simulink library "aerosimlib"  (Simulink 5.0)
values from neighbouring files (symbols this model uses):
  stdatm = [0 100 200 300 400 500 600 700 800 900 1000 1100 ... (4305 elements, 861x5)]    [stdatm.mat]
undefined symbols (not defined in the file or in its folder): AlphaBnd, b, BetaBnd, CDda, CDde, CDdf, CDdr, CDM, CDmin, CGempty, CGgross, CL0, CLa, CLalphadot, Clbeta, Clda, CLde, CLdf, Cldr, CLM, CLmind, Clp, CLq, Clr, Cm0, Cma, Cmalphadot, Cmde, Cmdf, CmM, Cmq, Cnbeta, Cnda, Cndr, Cnp, Cnr, CP, CT, CYbeta, CYda, CYdr, CYp, CYr, Displacement, dmy, Engine, EulerIni, FuelFlow, FuelIni, J, Jempty, Jeng, Jgross, Jprop, MAC, MAP, MAPLim, MassIni, MaxPower, mempty ... (+25)
libraries: aerosimlib x350, simulink3 x41
(part 8 of 10)

== system aerosimlib/FlightGear-Compatible/Complete Aircraft/CESSNA-182/Equations of Motion ==
  note: Inputs
  note: Outputs
  Accel : Inport  PortDimensions=[3 1]
  Moment : Inport  Port=2  PortDimensions=[3 1]
  Inertia : Inport  Port=3  PortDimensions=[4 1]
  Rearth : Inport  Port=4  PortDimensions=[2 1]
  Gravity : Inport  Port=5  PortDimensions=1
  AConGnd : Inport  Port=6  PortDimensions=1
  RST : Inport  Port=7  PortDimensions=1
  Angular Rate : aerosimlib/Equations of Motion/Geodetic-Frame EOM/Angular Rate  RatesIni=RatesIni
  Attitude (Quaternions) : aerosimlib/Equations of Motion/Body-Frame EOM/Kinematics (Quaternions)  QuaternionsIni=QuaternionsIni
  Body-Inertial DCM From Quaternions : aerosimlib/Transformations/Body-Inertial DCM From Quaternions
  Demux : Demux  Outputs=2
  Euler Angles From Quaternions : aerosimlib/Transformations/Euler Angles From Quaternions
  Position : aerosimlib/Equations of Motion/Geodetic-Frame EOM/Position  PositionIni=PositionIni
  Product : Product  Multiplication=Matrix(*)  SaturateOnIntegerOverflow=on  InputSameDT=on
  Velocity : aerosimlib/Equations of Motion/Geodetic-Frame EOM/Velocity  VelocitiesIni=VelocitiesIni
  VelB : Outport
  VelNED : Outport  Port=2
  Rates : Outport  Port=3
  Quaternions : Outport  Port=4
  Pos : Outport  Port=5
  DCM : Outport  Port=6
  Euler : Outport  Port=7
  Ang Acc : Outport  Port=8
  wires:
  Attitude (Quaternions)/1 -> Quaternions/1, Euler Angles From Quaternions/1, Body-Inertial DCM From Quaternions/1
  Position/1 -> Velocity/1, Angular Rate/3, Pos/1
  Position/2 -> Velocity/2, Angular Rate/4
  Velocity/1 -> Product/2, Position/1, VelNED/1
  Demux/1 -> Position/2
  Demux/2 -> Position/3
  Rearth/1 -> Demux/1
  Gravity/1 -> Velocity/5
  RST/1 -> Velocity/6, Position/5, Angular Rate/6, Attitude (Quaternions)/2
  Angular Rate/1 -> Rates/1, Attitude (Quaternions)/1
  Moment/1 -> Angular Rate/2
  Inertia/1 -> Angular Rate/1
  Body-Inertial DCM From Quaternions/1 -> Angular Rate/5, Velocity/4, Product/1, DCM/1
  AConGnd/1 -> Position/4
  Accel/1 -> Velocity/3
  Product/1 -> VelB/1
  Angular Rate/2 -> Ang Acc/1
  Euler Angles From Quaternions/1 -> Euler/1

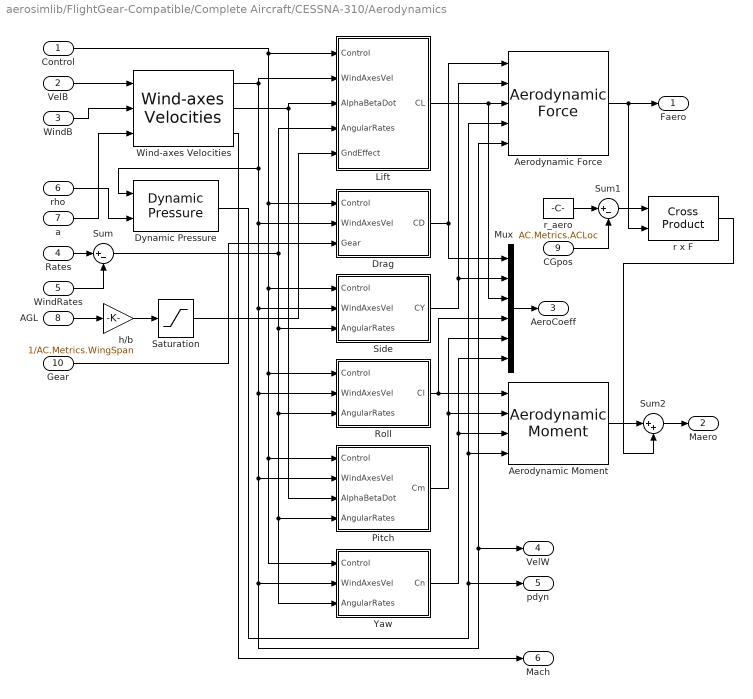
== system aerosimlib/FlightGear-Compatible/Complete Aircraft/CESSNA-310/Aerodynamics ==
  Control : Inport  PortDimensions=[4 1]
  VelB : Inport  Port=2  PortDimensions=[3 1]
  WindB : Inport  Port=3  PortDimensions=[3 1]
  Rates : Inport  Port=4  PortDimensions=[3 1]
  WindRates : Inport  Port=5  PortDimensions=[3 1]
  rho : Inport  Port=6  PortDimensions=1
  a : Inport  Port=7  PortDimensions=1
  AGL : Inport  Port=8  PortDimensions=1
  CGpos : Inport  Port=9  PortDimensions=[3 1]
  Gear : Inport  Port=10  PortDimensions=1
  Aerodynamic Force : aerosimlib/Aerodynamics/Aerodynamic Force  S=AC.Metrics.WingArea
  Aerodynamic Moment : aerosimlib/Aerodynamics/Aerodynamic Moment  c=AC.Metrics.WingChord  b=AC.Metrics.WingSpan  S=AC.Metrics.WingArea
  Drag : Subsystem
  Dynamic Pressure : aerosimlib/Aerodynamics/Dynamic Pressure
  Lift : Subsystem
  Mux : Mux  Inputs=6
  Pitch : Subsystem
  Roll : Subsystem
  Saturation : Saturate  UpperLimit=1  LowerLimit=0
  Side : Subsystem
  Sum : Sum  Inputs=|+-  SaturateOnIntegerOverflow=on  InputSameDT=on
  Sum1 : Sum  Inputs=|+-  SaturateOnIntegerOverflow=on  InputSameDT=on
  Sum2 : Sum  Inputs=|++  SaturateOnIntegerOverflow=on  InputSameDT=on
  Wind-axes Velocities : aerosimlib/Aerodynamics/Wind-axes Velocities  Vabnd=[0 1000]  betabnd=[-1 1]  alphabnd=AC.Aerodynamics.AlphaLim
  Yaw : Subsystem
  h/b : Gain  Gain=1/AC.Metrics.WingSpan  SaturateOnIntegerOverflow=on
  r x F : aerosimlib/Math/Cross Product
  r_aero : Constant  Value=AC.Metrics.ACLoc
  Faero : Outport
  Maero : Outport  Port=2
  AeroCoeff : Outport  Port=3
  VelW : Outport  Port=4
  pdyn : Outport  Port=5
  Mach : Outport  Port=6
  wires:
  Gear/1 -> Drag/3(Gear)
  r x F/1 -> Sum2/2
  Sum2/1 -> Maero/1
  Aerodynamic Moment/1 -> Sum2/1
  Sum1/1 -> r x F/1
  r_aero/1 -> Sum1/1
  CGpos/1 -> Sum1/2
  Rates/1 -> Sum/1
  Sum/1 -> Yaw/3(AngularRates), Pitch/4(AngularRates), Roll/3(AngularRates), Side/3(AngularRates), Lift/4(AngularRates)
  WindRates/1 -> Sum/2
  Saturation/1 -> Lift/5(GndEffect)
  AGL/1 -> h/b/1
  h/b/1 -> Saturation/1
  Wind-axes Velocities/3 -> Mach/1
  Aerodynamic Force/1 -> r x F/2, Faero/1
  Yaw/1(Cn) -> Mux/6, Aerodynamic Moment/3
  Pitch/1(Cm) -> Mux/5, Aerodynamic Moment/2
  Roll/1(Cl) -> Mux/4, Aerodynamic Moment/1
  Dynamic Pressure/1 -> pdyn/1, Aerodynamic Moment/4, Aerodynamic Force/4
  Side/1(CY) -> Mux/2, Aerodynamic Force/2
  Drag/1(CD) -> Mux/1, Aerodynamic Force/1
  Lift/1(CL) -> Mux/3, Aerodynamic Force/3
  Wind-axes Velocities/2 -> Lift/3(AlphaBetaDot), Pitch/3(AlphaBetaDot)
  Control/1 -> Pitch/1(Control), Yaw/1(Control), Roll/1(Control), Side/1(Control), Drag/1(Control), Lift/1(Control)
  Wind-axes Velocities/1 -> Lift/2(WindAxesVel), VelW/1, Aerodynamic Force/5, Yaw/2(WindAxesVel), Pitch/2(WindAxesVel), Roll/2(WindAxesVel), Side/2(WindAxesVel), Drag/2(WindAxesVel), Dynamic Pressure/1
  rho/1 -> Dynamic Pressure/2
  a/1 -> Wind-axes Velocities/3
  WindB/1 -> Wind-axes Velocities/2
  VelB/1 -> Wind-axes Velocities/1
  Mux/1 -> AeroCoeff/1

== system aerosimlib/FlightGear-Compatible/Complete Aircraft/CESSNA-310/Aircraft Inertia ==
  FuelFlow : Inport
  RST : Inport  Port=2
  1/Ntank : Gain  Gain=1/length(AC.Propulsion.Tank)  SaturateOnIntegerOverflow=on
  Empty Aircraft : aerosimlib/FlightGear-Compatible/Inertia/Empty Aircraft  Metrics=AC.Metrics
  Left Inner Tank : aerosimlib/FlightGear-Compatible/Propulsion/Tank/Fuel Tank  MassIni=FuelIni(3)  Tank=AC.Propulsion.Tank{3}
  Left Outer Tank : aerosimlib/FlightGear-Compatible/Propulsion/Tank/Fuel Tank  MassIni=FuelIni(1)  Tank=AC.Propulsion.Tank{1}
  Product{,1..3,5} (5 alike) : Product  SaturateOnIntegerOverflow=on  InputSameDT=on
  Product4 : Product  Inputs=*/  SaturateOnIntegerOverflow=on  InputSameDT=on
  Right Inner Tank : aerosimlib/FlightGear-Compatible/Propulsion/Tank/Fuel Tank  MassIni=FuelIni(4)  Tank=AC.Propulsion.Tank{4}
  Right Outer Tank : aerosimlib/FlightGear-Compatible/Propulsion/Tank/Fuel Tank  MassIni=FuelIni(2)  Tank=AC.Propulsion.Tank{2}
  Sum1 : Sum  Inputs=+++++  SaturateOnIntegerOverflow=on  InputSameDT=on
  Sum2 : Sum  Inputs=+++++  SaturateOnIntegerOverflow=on  InputSameDT=on
  Sum3 : Sum  Inputs=+++++  SaturateOnIntegerOverflow=on  InputSameDT=on
  Mass : Outport
  CG : Outport  Port=2
  Inertia : Outport  Port=3
  wires:
  Product5/1 -> Sum1/5
  Right Inner Tank/2 -> Product5/2
  Right Inner Tank/1 -> Sum2/5, Product5/1
  Right Inner Tank/3 -> Sum3/5
  Sum3/1 -> Inertia/1
  Left Inner Tank/3 -> Sum3/4
  Right Outer Tank/3 -> Sum3/3
  Left Outer Tank/3 -> Sum3/2
  Empty Aircraft/3 -> Sum3/1
  Product4/1 -> CG/1
  Sum1/1 -> Product4/1
  Product2/1 -> Sum1/4
  Product1/1 -> Sum1/3
  Product/1 -> Sum1/2
  Product3/1 -> Sum1/1
  Empty Aircraft/2 -> Product3/2
  Left Inner Tank/2 -> Product2/2
  Right Outer Tank/2 -> Product1/2
  Left Outer Tank/2 -> Product/2
  Left Inner Tank/1 -> Product2/1, Sum2/4
  Right Outer Tank/1 -> Product1/1, Sum2/3
  Left Outer Tank/1 -> Product/1, Sum2/2
  Empty Aircraft/1 -> Product3/1, Sum2/1
  Sum2/1 -> Product4/2, Mass/1
  RST/1 -> Left Outer Tank/2, Right Inner Tank/2, Left Inner Tank/2, Right Outer Tank/2
  FuelFlow/1 -> 1/Ntank/1
  1/Ntank/1 -> Right Inner Tank/1, Left Inner Tank/1, Left Outer Tank/1, Right Outer Tank/1

== system aerosimlib/FlightGear-Compatible/Complete Aircraft/CESSNA-310/Earth ==
  note: Inputs
  note: Outputs
  Position : Inport  PortDimensions=[3 1]  DataType=double
  EGM-96 : aerosimlib/Earth/EGM-96
  Ground Alt : Constant  Value=GndAlt
  Ground Detection : aerosimlib/Earth/Ground Detection
  Mux3 : Mux  Inputs=2
  WGS-84 : aerosimlib/Earth/WGS-84
  MSL : Outport
  AGL : Outport  Port=2
  AConGnd : Outport  Port=3
  Rearth : Outport  Port=4
  Requiv : Outport  Port=5
  Gravity : Outport  Port=6
  wires:
  Position/1 -> EGM-96/1, WGS-84/1
  Ground Alt/1 -> Ground Detection/2
  EGM-96/1 -> Ground Detection/1, MSL/1
  WGS-84/1 -> Mux3/1
  WGS-84/2 -> Mux3/2
  Ground Detection/2 -> AGL/1
  Ground Detection/1 -> AConGnd/1
  Mux3/1 -> Rearth/1
  WGS-84/3 -> Requiv/1
  WGS-84/4 -> Gravity/1

== system aerosimlib/FlightGear-Compatible/Complete Aircraft/CESSNA-310/Equations of Motion ==
  note: Inputs
  note: Outputs
  Accel : Inport  PortDimensions=[3 1]
  Moment : Inport  Port=2  PortDimensions=[3 1]
  Inertia : Inport  Port=3  PortDimensions=[4 1]
  Rearth : Inport  Port=4  PortDimensions=[2 1]
  Gravity : Inport  Port=5  PortDimensions=1
  AConGnd : Inport  Port=6  PortDimensions=1
  RST : Inport  Port=7  PortDimensions=1
  Angular Rate : aerosimlib/Equations of Motion/Geodetic-Frame EOM/Angular Rate  RatesIni=RatesIni
  Attitude (Quaternions) : aerosimlib/Equations of Motion/Body-Frame EOM/Kinematics (Quaternions)  QuaternionsIni=QuaternionsIni
  Body-Inertial DCM From Quaternions : aerosimlib/Transformations/Body-Inertial DCM From Quaternions
  Demux : Demux  Outputs=2
  Euler Angles From Quaternions : aerosimlib/Transformations/Euler Angles From Quaternions
  Position : aerosimlib/Equations of Motion/Geodetic-Frame EOM/Position  PositionIni=PositionIni
  Product : Product  Multiplication=Matrix(*)  SaturateOnIntegerOverflow=on  InputSameDT=on
  Velocity : aerosimlib/Equations of Motion/Geodetic-Frame EOM/Velocity  VelocitiesIni=VelocitiesIni
  VelB : Outport
  VelNED : Outport  Port=2
  Rates : Outport  Port=3
  Quaternions : Outport  Port=4
  Pos : Outport  Port=5
  DCM : Outport  Port=6
  Euler : Outport  Port=7
  Ang Acc : Outport  Port=8
  wires:
  Attitude (Quaternions)/1 -> Quaternions/1, Euler Angles From Quaternions/1, Body-Inertial DCM From Quaternions/1
  Position/1 -> Velocity/1, Angular Rate/3, Pos/1
  Position/2 -> Velocity/2, Angular Rate/4
  Velocity/1 -> Product/2, Position/1, VelNED/1
  Demux/1 -> Position/2
  Demux/2 -> Position/3
  Rearth/1 -> Demux/1
  Gravity/1 -> Velocity/5
  RST/1 -> Velocity/6, Position/5, Angular Rate/6, Attitude (Quaternions)/2
  Angular Rate/1 -> Rates/1, Attitude (Quaternions)/1
  Moment/1 -> Angular Rate/2
  Inertia/1 -> Angular Rate/1
  Body-Inertial DCM From Quaternions/1 -> Angular Rate/5, Velocity/4, Product/1, DCM/1
  AConGnd/1 -> Position/4
  Accel/1 -> Velocity/3
  Product/1 -> VelB/1
  Angular Rate/2 -> Ang Acc/1
  Euler Angles From Quaternions/1 -> Euler/1

== system aerosimlib/FlightGear-Compatible/Propulsion/Engine/Piston ==
  AirFlow Model : Subsystem  mask(AirFlow){VolEff=VolEff, Disp=Displacement}
      mask prompts: VolEff "Volumetric efficiency:"; Disp "Engine displacement"
      mask help: Estimate the airflow to a JSBSim engine as a function of MAP, RPM, and atmospheric conditions.
      mask Help:
      | Estimate the airflow to a JSBSim engine as a function of MAP, RPM, and atmospheric conditions.
      | <P><B>Inputs:</B>
      | <LI>MAP = the current manifold pressure</LI>
      | <LI>RPM = the current engine rotation speed</LI>
      | <LI>rho = the air density at current altitude</LI>
      | <LI>p = the current atmospheric pressure</LI>
      | </P>
      | <P><B>Outputs:</B>
      | <LI>Airflow = the mass airflow</LI>
      | </P>
      | <P><B>Parameters:</B>
      | <LI>Volumetric efficiency (approx. 0.8)</LI>
      | <LI>Engine displacement</LI>
      | </P>
  FG Piston Engine : Subsystem  mask(FlightGear Piston Engine){Eng=Engine, pSL=pSL, TSL=TSL}
      mask prompts: Eng "Engine structure:"; pSL "Sea-level pressure:"; TSL "Sea-level temperature:"
      mask help: The FlightGear Piston Engine computes the engine power output, air and fuel flow as functions of engine control settings and atmospheric conditions.
      mask Help:
      | The FlightGear Piston Engine computes the engine power output, air and fuel flow as functions of engine control settings and atmospheric conditions.
      | <P><B>Inputs:</B>
      | <LI>Thr = the current throttle fraction</LI>
      | <LI>Mix = the current air/fuel mixture setting</LI>
      | <LI>Omega = the current engine rotation speed</LI>
      | <LI>p = the atmospheric pressure</LI>
      | <LI>T = the outside-air temperature</LI>
      | <LI>rho = the air density at current altitude</LI>
      | </P>
      | <P><B>Outputs:</B>
      | <LI>MAP = the manifold pressure</LI>
      | <LI>AirFlow = the mass air flow</LI>
      | <LI>FuelFlow = the mass fuel flow</LI>
      | <LI>BSFC = the brake-specific fuel consumption</LI>
      | <LI>Power = the current power output</LI>
      | <LI>Torque = the torque delivered at engine shaft</LI>
      | </P>
      | <P><B>Parameters:</B>
      | <LI>Engine structure = a Matlab engine structure, which is part of the aircraft structure</LI>
      | <LI>The sea-level pressure and temperature for which the engine data is given.</LI>
      | </P>
  FuelFlow Model : Subsystem  mask(FuelFlow){pSL=pSL}
      mask prompts: pSL "Sea-level ambient pressure:"
      mask help: Estimate the mass fuel flow to the engine as a function of mixture setting, airflow, and atmospheric conditions.
      mask Help:
      | Estimate the mass fuel flow to the engine as a function of mixture setting, airflow, and atmospheric conditions.
      | <P><B>Inputs:</B>
      | <LI>Mix = the air/fuel mixture</LI>
      | <LI>p = the atmospheric pressure</LI>
      | <LI>AirFlow = the current mass airflow</LI>
      | </P>
      | <P><B>Outputs:</B>
      | <LI>EquivRatio = the equivalence ratio</LI>
      | <LI>FuelFlow = the mass fuel flow</LI>
      | </P>
      | <P><B>Parameters:</B>
      | <LI>Sea-level pressure</LI>
      | </P>
  Intake Model : Subsystem  mask(Intake){MAPLim=MAPLim, pSL=pSL}
      mask prompts: MAPLim "MAP limits:"; pSL "Sea-level ambient pressure:"
      mask help: The block computes the manifold pressure as a function of throttle area fraction, atmosphere parameters and fuel flow.
      mask Help:
      | The block computes the manifold pressure as a function of throttle area fraction, atmosphere parameters and fuel flow.
      | <P><B>Inputs:</B>
      | <LI>Thr = the current throttle fraction</LI>
      | <LI>p = the atmospheric pressure</LI>
      | </P>
      | <P><B>Outputs:</B>
      | <LI>MAP = the manifold pressure</LI>
      | </P>
      | <P><B>Parameters:</B>
      | <LI>MAP limits = the [min max] manifold pressure limits</LI>
      | <LI>Sea-level ambient pressure = the sea-level pressure for which the above MAP limits are given</LI>
      | </P>
  Power Model : Subsystem  mask(Power){TSL=TSL, MaxPower=MaxPower, Mixture=MixVec, PowerMixCor=PwrMixVec}
      mask prompts: TSL "Sea-level ambient temperature:"; MaxPower "Maximum power:"; Mixture "Mixture vector:"; PowerMixCor "Power-mixture correlation:"
      mask help: Estimate the power output of a JSBSim piston engine as a function of MAP, RPM, and propellant mass flow.
      mask Help:
      | Estimate the power output of a JSBSim piston engine as a function of MAP, RPM, and propellant mass flow.
      | <P><B>Inputs:</B>
      | <LI>MAP = the current manifold pressure</LI>
      | <LI>RPM = the current engine rotation speed</LI>
      | <LI>T = the outside air temperature</LI>
      | <LI>EquivRatio = the equivalence ratio</LI>
      | </P>
      | <P><B>Outputs:</B>
      | <LI>Power = the engine power output</LI>
      | </P>
      | <P><B>Parameters:</B>
      | <LI>Sea-level ambient temperature</LI>
      | <LI>Maximum power, at sea-level</LI>
      | <LI>Mixture vector = the mixture look-up table argument</LI>
      | <LI>Power-mixture correlation = look-up table for power-mixture correlation factor as a function of mixture</LI>
      | </P>

== system aerosimlib/FlightGear-Compatible/Propulsion/Tank/Fuel Tank ==
  MassFlow : Inport
  RST : Inport  Port=2
  2/5 : Constant  Value=2/5
  ChSign : Gain  Gain=-1  SaturateOnIntegerOverflow=on
  Flow Integrator : Integrator  ExternalReset=rising  InitialCondition=MassIni  LimitOutput=on  UpperSaturationLimit=Tank.Capacity  LowerSaturationLimit=0
  J : Product  Inputs=3  SaturateOnIntegerOverflow=on  InputSameDT=on
  J1 : Product  SaturateOnIntegerOverflow=on  InputSameDT=on
  J2 : Product  SaturateOnIntegerOverflow=on  InputSameDT=on
  J3 : Product  SaturateOnIntegerOverflow=on  InputSameDT=on
  Jxz : Product  Inputs=3  SaturateOnIntegerOverflow=on  InputSameDT=on
  Math Function{,1..3} (4 alike) : Math  Operator=square
  Mux : Mux  Inputs=3
  Mux1 : Mux
  Radius : Constant  Value=Tank.Radius
  Sum{,1..5} (6 alike) : Sum  SaturateOnIntegerOverflow=on  InputSameDT=on
  x pos : Constant  Value=Tank.Loc(1)
  y pos : Constant  Value=Tank.Loc(2)
  z pos : Constant  Value=Tank.Loc(3)
  Mass : Outport
  CG : Outport  Port=2
  Inertia : Outport  Port=3
  wires:
  Mux1/1 -> Inertia/1
  Jxz/1 -> Mux1/4
  Sum5/1 -> Mux1/3
  Sum4/1 -> Mux1/2
  Sum3/1 -> Mux1/1
  Mux/1 -> CG/1
  J3/1 -> Sum5/2
  J2/1 -> Sum4/2
  J1/1 -> Sum3/2
  J/1 -> Sum4/1, Sum5/1, Sum3/1
  Sum/1 -> J3/2
  Sum2/1 -> J2/2
  Sum1/1 -> J1/2
  Math Function3/1 -> Sum2/2, Sum1/2
  Math Function2/1 -> Sum1/1, Sum/2
  Math Function1/1 -> Sum2/1, Sum/1
  z pos/1 -> Math Function3/1, Mux/3, Jxz/3
  y pos/1 -> Mux/2, Math Function2/1
  x pos/1 -> Mux/1, Jxz/2, Math Function1/1
  Flow Integrator/1 -> Mass/1, J1/1, J2/1, J3/1, Jxz/1, J/1
  2/5/1 -> J/3
  Math Function/1 -> J/2
  Radius/1 -> Math Function/1
  RST/1 -> Flow Integrator/2
  MassFlow/1 -> ChSign/1
  ChSign/1 -> Flow Integrator/1

== system aerosimlib/FlightGear-Compatible/Propulsion/Thruster/Propeller ==
  FG Fixed-Pitch Propeller : Subsystem  mask(FG Fixed-pitch propeller model){Thr=Thruster}
      mask prompts: Thr "Thruster structure:"
      mask help: Fixed-pitch propeller model using look-up tables of thrust and power coefficients as functions of advance ratio.
      mask Help:
      | The block provides a fixed-pitch propeller model based on look-up tables for thrust and power coefficients as function of the advance ratio.
      | <P><B>Inputs:</B>
      | <LI>Airspeed = the current aircraft airspeed</LI>
      | <LI>rho = the air density at current aircraft altitude</LI>
      | <LI>Omega = the propeller rotation speed</LI>
      | </P>
      | <P><B>Output:</B>
      | <LI>Fprop = the thrust force generated by the propeller (on body x-axis)</LI>
      | <LI>Mprop = the moment generated by the propeller (on body x-axis)</LI>
      | <LI>PropCoeff = the 3x1 vector of propeller coefficients [J CT CP]</LI>
      | </P>
      | <P><B>Parameters:</B>
      | <LI>Thruster structure = the thruster structure which is a part of the Matlab structure</LI>
      | </P>
  FG Variable-Pitch Propeller : Subsystem  mask(FG Variable-pitch propeller model){Thr=Thr}
      mask prompts: Thr "Thruster structure:"
      mask help: Variable-pitch propeller model using look-up tables of thrust and power coefficients as functions of advance ratio and pitch angle.
      mask Help:
      | The block provides a variable-pitch propeller model based on look-up tables for thrust and power coefficients as function of the advance ratio and blade pitch angle.
      | <P><B>Inputs:</B>
      | <LI>Airspeed = the current aircraft airspeed</LI>
      | <LI>rho = the air density at current aircraft altitude</LI>
      | <LI>Omega = the propeller rotation speed</LI>
      | <LI>Pitch = the prop blade pitch angle</LI>
      | </P>
      | <P><B>Output:</B>
      | <LI>Fprop = the thrust force generated by the propeller (on body x-axis)</LI>
      | <LI>Mprop = the moment generated by the propeller (on body x-axis)</LI>
      | <LI>PropCoeff = the 3x1 vector of propeller coefficients [J CT CP]</LI>
      | </P>
      | <P><B>Parameters:</B>
      | <LI>Thruster structure = the thruster structure which is a part of the aircraft structure.</LI>
      | </P>

== system aerosimlib/Equations of Motion/Body-Frame EOM/Kinematics (Quaternions)/Normalization/Vector norm ==
  Vec : Inport
  Dot Product : simulink3/Math/Dot Product
  Math Function : Math  Operator=sqrt
  Mag : Outport
  wires:
  Math Function/1 -> Mag/1
  Dot Product/1 -> Math Function/1
  Vec/1 -> Dot Product/2, Dot Product/1

== system aerosimlib/FlightGear-Compatible/Complete Aircraft/CESSNA-172/Aerodynamics/Drag ==
  Control : Inport  PortDimensions=[4 1]
  WindAxesVel : Inport  Port=2  PortDimensions=[3 1]
  GndEffect : Inport  Port=3  PortDimensions=1
  CD alpha : Subsystem  BlockChoice=Table
      link override Table: Table=AC.Aerodynamics.Drag.Basic.CDwbh
      link override Value: Value=AC.Aerodynamics.Lift.Basic.kCLge
      link override Vector: Vector=AC.Aerodynamics.Lift.Basic.CLDf
      settings: AttributesFormatString=%<BlockChoice>  TemplateBlock=aerosimlib/FlightGear-Compatible/Aerodynamics/Coefficient  MemberBlocks=Table,Value,Vector
  CD beta : Subsystem  BlockChoice=Value
      link override Value: Value=AC.Aerodynamics.Drag.CDbeta
      settings: AttributesFormatString=%<BlockChoice>  TemplateBlock=aerosimlib/FlightGear-Compatible/Aerodynamics/Coefficient  MemberBlocks=Table,Value,Vector
  CD elevator : Subsystem  BlockChoice=Value
      link override Value: Value=AC.Aerodynamics.Drag.CDDe
      settings: AttributesFormatString=%<BlockChoice>  TemplateBlock=aerosimlib/FlightGear-Compatible/Aerodynamics/Coefficient  MemberBlocks=Table,Value,Vector
  CD flap : Subsystem  BlockChoice=Vector
      link override Value: Value=AC.Aerodynamics.Lift.Basic.kCLge
      link override Vector: Vector=AC.Aerodynamics.Drag.Basic.CDDf
      settings: AttributesFormatString=%<BlockChoice>  TemplateBlock=aerosimlib/FlightGear-Compatible/Aerodynamics/Coefficient  MemberBlocks=Table,Value,Vector
  CDo : Constant  Value=AC.Aerodynamics.Drag.CDo.Data
  Demux : Demux
  Demux1 : Demux  Outputs=3
  Product : Product  SaturateOnIntegerOverflow=on  InputSameDT=on
  Sum : Sum  SaturateOnIntegerOverflow=on  InputSameDT=on
  Sum1 : Sum  Inputs=++++  SaturateOnIntegerOverflow=on  InputSameDT=on
  Terminator : Terminator
  Terminator1 : Terminator
  Terminator5 : Terminator
  kCD ground effect : Subsystem  BlockChoice=Vector
      link override Value: Value=AC.Aerodynamics.Lift.Basic.kCLge
      link override Vector: Vector=AC.Aerodynamics.Drag.Basic.kCDge
      settings: AttributesFormatString=%<BlockChoice>  TemplateBlock=aerosimlib/FlightGear-Compatible/Aerodynamics/Coefficient  MemberBlocks=Table,Value,Vector
  CD : Outport
  wires:
  Demux/2 -> CD elevator/1(RowParam)
  WindAxesVel/1 -> Demux1/1
  Control/1 -> Demux/1
  Demux/1 -> CD alpha/2(ColParam), CD flap/1(RowParam)
  Demux/3 -> Terminator/1
  Demux/4 -> Terminator1/1
  Demux1/3 -> CD alpha/1(RowParam)
  CD alpha/1(Coeff) -> Sum/1
  CD flap/1(Coeff) -> Sum/2
  Sum/1 -> Product/1
  kCD ground effect/1(Coeff) -> Product/2
  Product/1 -> Sum1/1
  CDo/1 -> Sum1/2
  CD elevator/1(Coeff) -> Sum1/3
  CD beta/1(Coeff) -> Sum1/4
  Sum1/1 -> CD/1
  Demux1/1 -> Terminator5/1
  Demux1/2 -> CD beta/1(RowParam)
  GndEffect/1 -> kCD ground effect/1(RowParam)

== system aerosimlib/FlightGear-Compatible/Complete Aircraft/CESSNA-172/Aerodynamics/Lift ==
  Control : Inport  PortDimensions=[4 1]
  WindAxesVel : Inport  Port=2  PortDimensions=[3 1]
  AlphaBetaDot : Inport  Port=3  PortDimensions=[2 1]
  AngularRates : Inport  Port=4  PortDimensions=[3 1]
  HystParam : Inport  Port=5  PortDimensions=1
  GndEffect : Inport  Port=6  PortDimensions=1
  2 : Gain  Gain=2  SaturateOnIntegerOverflow=on
  CL alpha : Subsystem  BlockChoice=Table
      link override Table: Table=AC.Aerodynamics.Lift.Basic.CLwbh
      link override Value: Value=AC.Aerodynamics.Lift.Basic.kCLge
      link override Vector: Vector=AC.Aerodynamics.Lift.Basic.CLDf
      settings: AttributesFormatString=%<BlockChoice>  TemplateBlock=aerosimlib/FlightGear-Compatible/Aerodynamics/Coefficient  MemberBlocks=Table,Value,Vector
  CL elevator : Subsystem  BlockChoice=Value
      link override Value: Value=AC.Aerodynamics.Lift.CLDe
      settings: AttributesFormatString=%<BlockChoice>  TemplateBlock=aerosimlib/FlightGear-Compatible/Aerodynamics/Coefficient  MemberBlocks=Table,Value,Vector
  CL flap : Subsystem  BlockChoice=Vector
      link override Value: Value=AC.Aerodynamics.Lift.Basic.kCLge
      link override Vector: Vector=AC.Aerodynamics.Lift.Basic.CLDf
      settings: AttributesFormatString=%<BlockChoice>  TemplateBlock=aerosimlib/FlightGear-Compatible/Aerodynamics/Coefficient  MemberBlocks=Table,Value,Vector
  CL*c/(2V) : Product  Inputs=**/  SaturateOnIntegerOverflow=on  InputSameDT=on
  CLalphadot : Subsystem  BlockChoice=Value
      link override Value: Value=AC.Aerodynamics.Lift.CLadot
      settings: AttributesFormatString=%<BlockChoice>  TemplateBlock=aerosimlib/FlightGear-Compatible/Aerodynamics/Coefficient  MemberBlocks=Table,Value,Vector
  CLq : Subsystem  BlockChoice=Value
      link override Value: Value=AC.Aerodynamics.Lift.CLq
      settings: AttributesFormatString=%<BlockChoice>  TemplateBlock=aerosimlib/FlightGear-Compatible/Aerodynamics/Coefficient  MemberBlocks=Table,Value,Vector
  Demux : Demux
  Demux1 : Demux  Outputs=3
  Demux2 : Demux  Outputs=2
  Demux3 : Demux  Outputs=3
  Product : Product  SaturateOnIntegerOverflow=on  InputSameDT=on
  Sum : Sum  SaturateOnIntegerOverflow=on  InputSameDT=on
  Sum1 : Sum  Inputs=+++  SaturateOnIntegerOverflow=on  InputSameDT=on
  Sum2 : Sum  SaturateOnIntegerOverflow=on  InputSameDT=on
  Terminator{,1..4,6} (6 alike) : Terminator
  Wing chord : Constant  Value=AC.Metrics.WingChord
  kCL ground effect : Subsystem  BlockChoice=Vector
      link override Value: Value=AC.Aerodynamics.Lift.Basic.kCLge
      link override Vector: Vector=AC.Aerodynamics.Lift.Basic.kCLge
      settings: AttributesFormatString=%<BlockChoice>  TemplateBlock=aerosimlib/FlightGear-Compatible/Aerodynamics/Coefficient  MemberBlocks=Table,Value,Vector
  CL : Outport
  wires:
  CL*c/(2V)/1 -> Sum1/3
  CLq/1(Coeff) -> Sum2/2
  CLalphadot/1(Coeff) -> Sum2/1
  Sum2/1 -> CL*c/(2V)/1
  Wing chord/1 -> CL*c/(2V)/2
  2/1 -> CL*c/(2V)/3
  GndEffect/1 -> kCL ground effect/1(RowParam)
  HystParam/1 -> CL alpha/2(ColParam)
  Demux1/2 -> Terminator6/1
  Demux1/1 -> 2/1
  Sum1/1 -> CL/1
  CL elevator/1(Coeff) -> Sum1/2
  Product/1 -> Sum1/1
  kCL ground effect/1(Coeff) -> Product/2
  Sum/1 -> Product/1
  CL flap/1(Coeff) -> Sum/2
  CL alpha/1(Coeff) -> Sum/1
  Demux3/3 -> Terminator4/1
  Demux3/1 -> Terminator3/1
  Demux2/2 -> Terminator2/1
  Demux3/2 -> CLq/1(RowParam)
  Demux2/1 -> CLalphadot/1(RowParam)
  Demux1/3 -> CL alpha/1(RowParam)
  Demux/4 -> Terminator1/1
  Demux/3 -> Terminator/1
  Demux/2 -> CL elevator/1(RowParam)
  Demux/1 -> CL flap/1(RowParam)
  AngularRates/1 -> Demux3/1
  AlphaBetaDot/1 -> Demux2/1
  Control/1 -> Demux/1
  WindAxesVel/1 -> Demux1/1

== system aerosimlib/FlightGear-Compatible/Complete Aircraft/CESSNA-172/Aerodynamics/Pitch ==
  Control : Inport  PortDimensions=[4 1]
  WindAxesVel : Inport  Port=2  PortDimensions=[3 1]
  AlphaBetaDot : Inport  Port=3  PortDimensions=[2 1]
  AngularRates : Inport  Port=4  PortDimensions=[3 1]
  2 : Gain  Gain=2  SaturateOnIntegerOverflow=on
  Cm alpha : Subsystem  BlockChoice=Value
      link override Table: Table=AC.Aerodynamics.Lift.Basic.CLwbh
      link override Value: Value=AC.Aerodynamics.Pitch.Cmalpha
      link override Vector: Vector=AC.Aerodynamics.Lift.Basic.CLDf
      settings: AttributesFormatString=%<BlockChoice>  TemplateBlock=aerosimlib/FlightGear-Compatible/Aerodynamics/Coefficient  MemberBlocks=Table,Value,Vector
  Cm elevator : Subsystem  BlockChoice=Value
      link override Value: Value=AC.Aerodynamics.Pitch.Cmde
      settings: AttributesFormatString=%<BlockChoice>  TemplateBlock=aerosimlib/FlightGear-Compatible/Aerodynamics/Coefficient  MemberBlocks=Table,Value,Vector
  Cm flap : Subsystem  BlockChoice=Vector
      link override Value: Value=AC.Aerodynamics.Lift.Basic.kCLge
      link override Vector: Vector=AC.Aerodynamics.Pitch.Cmdf
      settings: AttributesFormatString=%<BlockChoice>  TemplateBlock=aerosimlib/FlightGear-Compatible/Aerodynamics/Coefficient  MemberBlocks=Table,Value,Vector
  Cm*c/(2V) : Product  Inputs=**/  SaturateOnIntegerOverflow=on  InputSameDT=on
  Cmalphadot : Subsystem  BlockChoice=Value
      link override Value: Value=AC.Aerodynamics.Pitch.Cmadot
      settings: AttributesFormatString=%<BlockChoice>  TemplateBlock=aerosimlib/FlightGear-Compatible/Aerodynamics/Coefficient  MemberBlocks=Table,Value,Vector
  Cmo : Constant  Value=AC.Aerodynamics.Pitch.Cmo.Data
  Cmq : Subsystem  BlockChoice=Value
      link override Value: Value=AC.Aerodynamics.Pitch.Cmq
      settings: AttributesFormatString=%<BlockChoice>  TemplateBlock=aerosimlib/FlightGear-Compatible/Aerodynamics/Coefficient  MemberBlocks=Table,Value,Vector
  Demux : Demux
  Demux1 : Demux  Outputs=3
  Demux2 : Demux  Outputs=2
  Demux3 : Demux  Outputs=3
  Sum1 : Sum  Inputs=+++++  SaturateOnIntegerOverflow=on  InputSameDT=on
  Sum2 : Sum  SaturateOnIntegerOverflow=on  InputSameDT=on
  Terminator{,1..4,6} (6 alike) : Terminator
  Wing chord : Constant  Value=AC.Metrics.WingChord
  Cm : Outport
  wires:
  Cm*c/(2V)/1 -> Sum1/5
  Cm elevator/1(Coeff) -> Sum1/4
  Cmo/1 -> Sum1/3
  Cm flap/1(Coeff) -> Sum1/2
  Cm alpha/1(Coeff) -> Sum1/1
  Demux3/2 -> Cmq/1(RowParam)
  Demux2/1 -> Cmalphadot/1(RowParam)
  Demux1/3 -> Cm alpha/1(RowParam)
  Demux1/1 -> 2/1
  Demux/2 -> Cm elevator/1(RowParam)
  Demux/1 -> Cm flap/1(RowParam)
  WindAxesVel/1 -> Demux1/1
  Control/1 -> Demux/1
  AlphaBetaDot/1 -> Demux2/1
  AngularRates/1 -> Demux3/1
  Demux/3 -> Terminator/1
  Demux/4 -> Terminator1/1
  Demux2/2 -> Terminator2/1
  Demux3/1 -> Terminator3/1
  Demux3/3 -> Terminator4/1
  Sum1/1 -> Cm/1
  Demux1/2 -> Terminator6/1
  2/1 -> Cm*c/(2V)/3
  Wing chord/1 -> Cm*c/(2V)/2
  Sum2/1 -> Cm*c/(2V)/1
  Cmalphadot/1(Coeff) -> Sum2/1
  Cmq/1(Coeff) -> Sum2/2

== system aerosimlib/FlightGear-Compatible/Complete Aircraft/CESSNA-172/Aerodynamics/Roll ==
  Control : Inport  PortDimensions=[4 1]
  WindAxesVel : Inport  Port=2  PortDimensions=[3 1]
  AngularRates : Inport  Port=3  PortDimensions=[3 1]
  2 : Gain  Gain=2  SaturateOnIntegerOverflow=on
  Cl aileron : Subsystem  BlockChoice=Value
      link override Value: Value=AC.Aerodynamics.Roll.ClDa
      settings: AttributesFormatString=%<BlockChoice>  TemplateBlock=aerosimlib/FlightGear-Compatible/Aerodynamics/Coefficient  MemberBlocks=Table,Value,Vector
  Cl beta : Subsystem  BlockChoice=Vector
      link override Value: Value=AC.Aerodynamics.Lift.Basic.kCLge
      link override Vector: Vector=AC.Aerodynamics.Roll.Clb
      settings: AttributesFormatString=%<BlockChoice>  TemplateBlock=aerosimlib/FlightGear-Compatible/Aerodynamics/Coefficient  MemberBlocks=Table,Value,Vector
  Cl rudder : Subsystem  BlockChoice=Value
      link override Value: Value=AC.Aerodynamics.Roll.Cldr
      settings: AttributesFormatString=%<BlockChoice>  TemplateBlock=aerosimlib/FlightGear-Compatible/Aerodynamics/Coefficient  MemberBlocks=Table,Value,Vector
  Cl*b/(2V) : Product  Inputs=**/  SaturateOnIntegerOverflow=on  InputSameDT=on
  Clp : Subsystem  BlockChoice=Value
      link override Value: Value=AC.Aerodynamics.Roll.Clp
      settings: AttributesFormatString=%<BlockChoice>  TemplateBlock=aerosimlib/FlightGear-Compatible/Aerodynamics/Coefficient  MemberBlocks=Table,Value,Vector
  Clr : Subsystem  BlockChoice=Table
      link override Table: Table=AC.Aerodynamics.Roll.Clr
      link override Value: Value=AC.Aerodynamics.Side.CYdr
      link override Vector: Vector=AC.Aerodynamics.Roll.Clr
      settings: AttributesFormatString=%<BlockChoice>  TemplateBlock=aerosimlib/FlightGear-Compatible/Aerodynamics/Coefficient  MemberBlocks=Table,Value,Vector
  Clr*r : Product  SaturateOnIntegerOverflow=on  InputSameDT=on
  Demux : Demux
  Demux1 : Demux  Outputs=3
  Demux3 : Demux  Outputs=3
  Sum : Sum  SaturateOnIntegerOverflow=on  InputSameDT=on
  Sum1 : Sum  Inputs=++++  SaturateOnIntegerOverflow=on  InputSameDT=on
  Terminator3 : Terminator
  Terminator4 : Terminator
  Wing span : Constant  Value=AC.Metrics.WingSpan
  Cl : Outport
  wires:
  Sum1/1 -> Cl/1
  AngularRates/1 -> Demux3/1
  Control/1 -> Demux/1
  WindAxesVel/1 -> Demux1/1
  Clp/1(Coeff) -> Sum/1
  Wing span/1 -> Cl*b/(2V)/2
  2/1 -> Cl*b/(2V)/3
  Sum/1 -> Cl*b/(2V)/1
  Demux1/1 -> 2/1
  Demux1/2 -> Cl beta/1(RowParam)
  Demux/3 -> Cl aileron/1(RowParam)
  Demux/4 -> Cl rudder/1(RowParam)
  Demux3/1 -> Clp/1(RowParam)
  Demux3/2 -> Terminator4/1
  Demux1/3 -> Clr/1(RowParam)
  Demux/1 -> Clr/2(ColParam)
  Demux/2 -> Terminator3/1
  Cl beta/1(Coeff) -> Sum1/1
  Cl aileron/1(Coeff) -> Sum1/2
  Cl rudder/1(Coeff) -> Sum1/3
  Cl*b/(2V)/1 -> Sum1/4
  Clr*r/1 -> Sum/2
  Clr/1(Coeff) -> Clr*r/1
  Demux3/3 -> Clr*r/2

== system aerosimlib/FlightGear-Compatible/Complete Aircraft/CESSNA-172/Aerodynamics/Side ==
  Control : Inport  PortDimensions=[4 1]
  WindAxesVel : Inport  Port=2  PortDimensions=[3 1]
  AngularRates : Inport  Port=3  PortDimensions=[3 1]
  2 : Gain  Gain=2  SaturateOnIntegerOverflow=on
  CY aileron : Subsystem  BlockChoice=Value
      link override Value: Value=AC.Aerodynamics.Side.CYda
      settings: AttributesFormatString=%<BlockChoice>  TemplateBlock=aerosimlib/FlightGear-Compatible/Aerodynamics/Coefficient  MemberBlocks=Table,Value,Vector
  CY beta : Subsystem  BlockChoice=Table
      link override Table: Table=AC.Aerodynamics.Side.CYb
      link override Value: Value=AC.Aerodynamics.Lift.Basic.kCLge
      link override Vector: Vector=AC.Aerodynamics.Side.CYb
      settings: AttributesFormatString=%<BlockChoice>  TemplateBlock=aerosimlib/FlightGear-Compatible/Aerodynamics/Coefficient  MemberBlocks=Table,Value,Vector
  CY rudder : Subsystem  BlockChoice=Value
      link override Value: Value=AC.Aerodynamics.Side.CYdr
      settings: AttributesFormatString=%<BlockChoice>  TemplateBlock=aerosimlib/FlightGear-Compatible/Aerodynamics/Coefficient  MemberBlocks=Table,Value,Vector
  CY*b/(2V) : Product  Inputs=**/  SaturateOnIntegerOverflow=on  InputSameDT=on
  CYp : Subsystem  BlockChoice=Table
      link override Table: Table=AC.Aerodynamics.Side.CYp
      link override Value: Value=AC.Aerodynamics.Side.CYp
      settings: AttributesFormatString=%<BlockChoice>  TemplateBlock=aerosimlib/FlightGear-Compatible/Aerodynamics/Coefficient  MemberBlocks=Table,Value,Vector
  CYr : Subsystem  BlockChoice=Table
      link override Table: Table=AC.Aerodynamics.Side.CYr
      link override Value: Value=AC.Aerodynamics.Side.CYr
      settings: AttributesFormatString=%<BlockChoice>  TemplateBlock=aerosimlib/FlightGear-Compatible/Aerodynamics/Coefficient  MemberBlocks=Table,Value,Vector
  Demux : Demux
  Demux1 : Demux  Outputs=3
  Demux3 : Demux  Outputs=3
  Product : Product  SaturateOnIntegerOverflow=on  InputSameDT=on
  Product1 : Product  SaturateOnIntegerOverflow=on  InputSameDT=on
  Sum : Sum  SaturateOnIntegerOverflow=on  InputSameDT=on
  Sum1 : Sum  Inputs=++++  SaturateOnIntegerOverflow=on  InputSameDT=on
  Terminator3 : Terminator
  Terminator4 : Terminator
  Wing span : Constant  Value=AC.Metrics.WingSpan
  CY : Outport
  wires:
  CY*b/(2V)/1 -> Sum1/4
  CY rudder/1(Coeff) -> Sum1/3
  CY aileron/1(Coeff) -> Sum1/2
  CY beta/1(Coeff) -> Sum1/1
  Demux/2 -> Terminator3/1
  Demux/1 -> CY beta/2(ColParam), CYp/2(ColParam), CYr/2(ColParam)
  Demux1/3 -> CYp/1(RowParam), CYr/1(RowParam)
  Demux3/2 -> Terminator4/1
  Demux/4 -> CY rudder/1(RowParam)
  Demux/3 -> CY aileron/1(RowParam)
  Demux1/2 -> CY beta/1(RowParam)
  Demux1/1 -> 2/1
  Sum/1 -> CY*b/(2V)/1
  2/1 -> CY*b/(2V)/3
  Wing span/1 -> CY*b/(2V)/2
  WindAxesVel/1 -> Demux1/1
  Control/1 -> Demux/1
  AngularRates/1 -> Demux3/1
  Sum1/1 -> CY/1
  Product/1 -> Sum/1
  Product1/1 -> Sum/2
  CYp/1(Coeff) -> Product/1
  CYr/1(Coeff) -> Product1/1
  Demux3/1 -> Product/2
  Demux3/3 -> Product1/2

== system aerosimlib/FlightGear-Compatible/Complete Aircraft/CESSNA-172/Aerodynamics/Yaw ==
  Control : Inport  PortDimensions=[4 1]
  WindAxesVel : Inport  Port=2  PortDimensions=[3 1]
  AngularRates : Inport  Port=3  PortDimensions=[3 1]
  2 : Gain  Gain=2  SaturateOnIntegerOverflow=on
  Cn aileron : Subsystem  BlockChoice=Value
      link override Value: Value=AC.Aerodynamics.Yaw.Cnda
      settings: AttributesFormatString=%<BlockChoice>  TemplateBlock=aerosimlib/FlightGear-Compatible/Aerodynamics/Coefficient  MemberBlocks=Table,Value,Vector
  Cn beta : Subsystem  BlockChoice=Vector
      link override Value: Value=AC.Aerodynamics.Lift.Basic.kCLge
      link override Vector: Vector=AC.Aerodynamics.Yaw.Cnb
      settings: AttributesFormatString=%<BlockChoice>  TemplateBlock=aerosimlib/FlightGear-Compatible/Aerodynamics/Coefficient  MemberBlocks=Table,Value,Vector
  Cn rudder : Subsystem  BlockChoice=Value
      link override Value: Value=AC.Aerodynamics.Yaw.Cndr
      settings: AttributesFormatString=%<BlockChoice>  TemplateBlock=aerosimlib/FlightGear-Compatible/Aerodynamics/Coefficient  MemberBlocks=Table,Value,Vector
  Cn*b/(2V) : Product  Inputs=**/  SaturateOnIntegerOverflow=on  InputSameDT=on
  Cnp : Subsystem  BlockChoice=Value
      link override Value: Value=AC.Aerodynamics.Yaw.Cnp
      settings: AttributesFormatString=%<BlockChoice>  TemplateBlock=aerosimlib/FlightGear-Compatible/Aerodynamics/Coefficient  MemberBlocks=Table,Value,Vector
  Cnr : Subsystem  BlockChoice=Value
      link override Value: Value=AC.Aerodynamics.Yaw.Cnr
      link override Vector: Vector=AC.Aerodynamics.Roll.Clr
      settings: AttributesFormatString=%<BlockChoice>  TemplateBlock=aerosimlib/FlightGear-Compatible/Aerodynamics/Coefficient  MemberBlocks=Table,Value,Vector
  Demux : Demux
  Demux1 : Demux  Outputs=3
  Demux3 : Demux  Outputs=3
  Sum : Sum  SaturateOnIntegerOverflow=on  InputSameDT=on
  Sum1 : Sum  Inputs=++++  SaturateOnIntegerOverflow=on  InputSameDT=on
  Terminator{1..4} (4 alike) : Terminator
  Wing span : Constant  Value=AC.Metrics.WingSpan
  Cn : Outport
  wires:
  Cn*b/(2V)/1 -> Sum1/4
  Cn rudder/1(Coeff) -> Sum1/3
  Cn aileron/1(Coeff) -> Sum1/2
  Cn beta/1(Coeff) -> Sum1/1
  Demux/2 -> Terminator3/1
  Demux/1 -> Terminator2/1
  Demux1/3 -> Terminator1/1
  Demux3/2 -> Terminator4/1
  Demux3/3 -> Cnr/1(RowParam)
  Demux3/1 -> Cnp/1(RowParam)
  Demux/4 -> Cn rudder/1(RowParam)
  Demux/3 -> Cn aileron/1(RowParam)
  Demux1/2 -> Cn beta/1(RowParam)
  Demux1/1 -> 2/1
  Sum/1 -> Cn*b/(2V)/1
  2/1 -> Cn*b/(2V)/3
  Wing span/1 -> Cn*b/(2V)/2
  Cnr/1(Coeff) -> Sum/2
  Cnp/1(Coeff) -> Sum/1
  WindAxesVel/1 -> Demux1/1
  Control/1 -> Demux/1
  AngularRates/1 -> Demux3/1
  Sum1/1 -> Cn/1

== system aerosimlib/FlightGear-Compatible/Complete Aircraft/CESSNA-182/Aerodynamics/Drag ==
  Control : Inport  PortDimensions=[4 1]
  WindAxesVel : Inport  Port=2  PortDimensions=[3 1]
  CD alpha : Subsystem  BlockChoice=Vector
      link override Table: Table=AC.Aerodynamics.Drag.Basic.CDwbh
      link override Value: Value=AC.Aerodynamics.Lift.Basic.kCLge
      link override Vector: Vector=AC.Aerodynamics.Drag.CDalpha
      settings: AttributesFormatString=%<BlockChoice>  TemplateBlock=aerosimlib/FlightGear-Compatible/Aerodynamics/Coefficient  MemberBlocks=Table,Value,Vector
  CD beta : Subsystem  BlockChoice=Value
      link override Value: Value=AC.Aerodynamics.Drag.CDbeta
      settings: AttributesFormatString=%<BlockChoice>  TemplateBlock=aerosimlib/FlightGear-Compatible/Aerodynamics/Coefficient  MemberBlocks=Table,Value,Vector
  CD elevator : Subsystem  BlockChoice=Value
      link override Value: Value=AC.Aerodynamics.Drag.CDDe
      settings: AttributesFormatString=%<BlockChoice>  TemplateBlock=aerosimlib/FlightGear-Compatible/Aerodynamics/Coefficient  MemberBlocks=Table,Value,Vector
  CD flap : Subsystem  BlockChoice=Table
      link override Table: Table=AC.Aerodynamics.Drag.CDDf
      link override Value: Value=AC.Aerodynamics.Lift.Basic.kCLge
      link override Vector: Vector=AC.Aerodynamics.Drag.Basic.CDDf
      settings: AttributesFormatString=%<BlockChoice>  TemplateBlock=aerosimlib/FlightGear-Compatible/Aerodynamics/Coefficient  MemberBlocks=Table,Value,Vector
  CDo : Constant  Value=AC.Aerodynamics.Drag.CDo.Data
  Demux : Demux
  Demux1 : Demux  Outputs=3
  Sum : Sum  SaturateOnIntegerOverflow=on  InputSameDT=on
  Sum1 : Sum  Inputs=++++  SaturateOnIntegerOverflow=on  InputSameDT=on
  Terminator : Terminator
  Terminator1 : Terminator
  Terminator5 : Terminator
  CD : Outport
  wires:
  Demux/1 -> CD flap/2(ColParam)
  Demux/2 -> CD elevator/1(RowParam)
  WindAxesVel/1 -> Demux1/1
  Control/1 -> Demux/1
  Demux/3 -> Terminator/1
  Demux/4 -> Terminator1/1
  Demux1/3 -> CD flap/1(RowParam), CD alpha/1(RowParam)
  CD alpha/1(Coeff) -> Sum/1
  CD flap/1(Coeff) -> Sum/2
  Sum/1 -> Sum1/1
  CDo/1 -> Sum1/2
  CD elevator/1(Coeff) -> Sum1/3
  CD beta/1(Coeff) -> Sum1/4
  Sum1/1 -> CD/1
  Demux1/1 -> Terminator5/1
  Demux1/2 -> CD beta/1(RowParam)

== system aerosimlib/FlightGear-Compatible/Complete Aircraft/CESSNA-182/Aerodynamics/Lift ==
  Control : Inport  PortDimensions=[4 1]
  WindAxesVel : Inport  Port=2  PortDimensions=[3 1]
  AlphaBetaDot : Inport  Port=3  PortDimensions=[2 1]
  AngularRates : Inport  Port=4  PortDimensions=[3 1]
  GndEffect : Inport  Port=5  PortDimensions=1
  2 : Gain  Gain=2  SaturateOnIntegerOverflow=on
  CL alpha : Subsystem  BlockChoice=Vector
      link override Table: Table=AC.Aerodynamics.Lift.Basic.CLalpha
      link override Value: Value=AC.Aerodynamics.Lift.Basic.kCLge
      link override Vector: Vector=AC.Aerodynamics.Lift.Basic.CLalpha
      settings: AttributesFormatString=%<BlockChoice>  TemplateBlock=aerosimlib/FlightGear-Compatible/Aerodynamics/Coefficient  MemberBlocks=Table,Value,Vector
  CL elevator : Subsystem  BlockChoice=Value
      link override Value: Value=AC.Aerodynamics.Lift.CLDe
      settings: AttributesFormatString=%<BlockChoice>  TemplateBlock=aerosimlib/FlightGear-Compatible/Aerodynamics/Coefficient  MemberBlocks=Table,Value,Vector
  CL flap : Subsystem  BlockChoice=Vector
      link override Value: Value=AC.Aerodynamics.Lift.Basic.kCLge
      link override Vector: Vector=AC.Aerodynamics.Lift.Basic.CLDf
      settings: AttributesFormatString=%<BlockChoice>  TemplateBlock=aerosimlib/FlightGear-Compatible/Aerodynamics/Coefficient  MemberBlocks=Table,Value,Vector
  CL*c/(2V) : Product  Inputs=**/  SaturateOnIntegerOverflow=on  InputSameDT=on
  CLalphadot : Subsystem  BlockChoice=Value
      link override Value: Value=AC.Aerodynamics.Lift.CLadot
      settings: AttributesFormatString=%<BlockChoice>  TemplateBlock=aerosimlib/FlightGear-Compatible/Aerodynamics/Coefficient  MemberBlocks=Table,Value,Vector
  CLo : Constant  Value=AC.Aerodynamics.Lift.Basic.CLo.Data
  CLq : Subsystem  BlockChoice=Value
      link override Value: Value=AC.Aerodynamics.Lift.CLq
      settings: AttributesFormatString=%<BlockChoice>  TemplateBlock=aerosimlib/FlightGear-Compatible/Aerodynamics/Coefficient  MemberBlocks=Table,Value,Vector
  Demux : Demux
  Demux1 : Demux  Outputs=3
  Demux2 : Demux  Outputs=2
  Demux3 : Demux  Outputs=3
  Product : Product  SaturateOnIntegerOverflow=on  InputSameDT=on
  Sum : Sum  Inputs=+++  SaturateOnIntegerOverflow=on  InputSameDT=on
  Sum1 : Sum  Inputs=+++  SaturateOnIntegerOverflow=on  InputSameDT=on
  Sum2 : Sum  SaturateOnIntegerOverflow=on  InputSameDT=on
  Terminator{,1..4,6} (6 alike) : Terminator
  Wing chord : Constant  Value=AC.Metrics.WingChord
  kCL ground effect : Subsystem  BlockChoice=Vector
      link override Value: Value=AC.Aerodynamics.Lift.Basic.kCLge
      link override Vector: Vector=AC.Aerodynamics.Lift.Basic.kCLge
      settings: AttributesFormatString=%<BlockChoice>  TemplateBlock=aerosimlib/FlightGear-Compatible/Aerodynamics/Coefficient  MemberBlocks=Table,Value,Vector
  CL : Outport
  wires:
  CLo/1 -> Sum/3
  CL*c/(2V)/1 -> Sum1/3
  CLq/1(Coeff) -> Sum2/2
  CLalphadot/1(Coeff) -> Sum2/1
  Sum2/1 -> CL*c/(2V)/1
  Wing chord/1 -> CL*c/(2V)/2
  2/1 -> CL*c/(2V)/3
  GndEffect/1 -> kCL ground effect/1(RowParam)
  Demux1/2 -> Terminator6/1
  Demux1/1 -> 2/1
  Sum1/1 -> CL/1
  CL elevator/1(Coeff) -> Sum1/2
  Product/1 -> Sum1/1
  kCL ground effect/1(Coeff) -> Product/2
  Sum/1 -> Product/1
  CL flap/1(Coeff) -> Sum/2
  CL alpha/1(Coeff) -> Sum/1
  Demux3/3 -> Terminator4/1
  Demux3/1 -> Terminator3/1
  Demux2/2 -> Terminator2/1
  Demux3/2 -> CLq/1(RowParam)
  Demux2/1 -> CLalphadot/1(RowParam)
  Demux1/3 -> CL alpha/1(RowParam)
  Demux/4 -> Terminator1/1
  Demux/3 -> Terminator/1
  Demux/2 -> CL elevator/1(RowParam)
  Demux/1 -> CL flap/1(RowParam)
  AngularRates/1 -> Demux3/1
  AlphaBetaDot/1 -> Demux2/1
  Control/1 -> Demux/1
  WindAxesVel/1 -> Demux1/1

== system aerosimlib/FlightGear-Compatible/Complete Aircraft/CESSNA-182/Aerodynamics/Pitch ==
  Control : Inport  PortDimensions=[4 1]
  WindAxesVel : Inport  Port=2  PortDimensions=[3 1]
  AlphaBetaDot : Inport  Port=3  PortDimensions=[2 1]
  AngularRates : Inport  Port=4  PortDimensions=[3 1]
  2 : Gain  Gain=2  SaturateOnIntegerOverflow=on
  Cm alpha : Subsystem  BlockChoice=Vector
      link override Table: Table=AC.Aerodynamics.Lift.Basic.CLwbh
      link override Value: Value=AC.Aerodynamics.Pitch.Cmalpha
      link override Vector: Vector=AC.Aerodynamics.Pitch.Cmalpha
      settings: AttributesFormatString=%<BlockChoice>  TemplateBlock=aerosimlib/FlightGear-Compatible/Aerodynamics/Coefficient  MemberBlocks=Table,Value,Vector
  Cm elevator : Subsystem  BlockChoice=Vector
      link override Value: Value=AC.Aerodynamics.Pitch.CmDe
      link override Vector: Vector=AC.Aerodynamics.Pitch.CmDe
      settings: AttributesFormatString=%<BlockChoice>  TemplateBlock=aerosimlib/FlightGear-Compatible/Aerodynamics/Coefficient  MemberBlocks=Table,Value,Vector
  Cm flap : Subsystem  BlockChoice=Vector
      link override Value: Value=AC.Aerodynamics.Lift.Basic.kCLge
      link override Vector: Vector=AC.Aerodynamics.Pitch.CmDf
      settings: AttributesFormatString=%<BlockChoice>  TemplateBlock=aerosimlib/FlightGear-Compatible/Aerodynamics/Coefficient  MemberBlocks=Table,Value,Vector
  Cm*c/(2V) : Product  Inputs=**/  SaturateOnIntegerOverflow=on  InputSameDT=on
  Cma*a : Product  SaturateOnIntegerOverflow=on  InputSameDT=on
  Cma*a1 : Product  SaturateOnIntegerOverflow=on  InputSameDT=on
  Cma*a2 : Product  SaturateOnIntegerOverflow=on  InputSameDT=on
  Cmalphadot : Subsystem  BlockChoice=Vector
      link override Value: Value=AC.Aerodynamics.Pitch.Cmadot
      link override Vector: Vector=AC.Aerodynamics.Pitch.Cmadot
      settings: AttributesFormatString=%<BlockChoice>  TemplateBlock=aerosimlib/FlightGear-Compatible/Aerodynamics/Coefficient  MemberBlocks=Table,Value,Vector
  Cmo : Constant  Value=AC.Aerodynamics.Pitch.Cmo.Data
  Cmq : Subsystem  BlockChoice=Value
      link override Value: Value=AC.Aerodynamics.Pitch.Cmq
      settings: AttributesFormatString=%<BlockChoice>  TemplateBlock=aerosimlib/FlightGear-Compatible/Aerodynamics/Coefficient  MemberBlocks=Table,Value,Vector
  Demux : Demux
  Demux1 : Demux  Outputs=3
  Demux2 : Demux  Outputs=2
  Demux3 : Demux  Outputs=3
  Sum1 : Sum  Inputs=+++++  SaturateOnIntegerOverflow=on  InputSameDT=on
  Sum2 : Sum  SaturateOnIntegerOverflow=on  InputSameDT=on
  Terminator{,1..4,6} (6 alike) : Terminator
  Wing chord : Constant  Value=AC.Metrics.WingChord
  Cm : Outport
  wires:
  Cma*a2/1 -> Sum1/4
  Cm elevator/1(Coeff) -> Cma*a2/2
  Demux/2 -> Cma*a2/1
  Demux2/1 -> Cma*a1/2
  Cmalphadot/1(Coeff) -> Cma*a1/1
  Cma*a1/1 -> Sum2/1
  Cm alpha/1(Coeff) -> Cma*a/1
  Cma*a/1 -> Sum1/1
  Cm*c/(2V)/1 -> Sum1/5
  Cmo/1 -> Sum1/3
  Cm flap/1(Coeff) -> Sum1/2
  Demux3/2 -> Cmq/1(RowParam)
  Demux1/3 -> Cm elevator/1(RowParam), Cmalphadot/1(RowParam), Cma*a/2, Cm alpha/1(RowParam)
  Demux1/1 -> 2/1
  Demux/1 -> Cm flap/1(RowParam)
  WindAxesVel/1 -> Demux1/1
  Control/1 -> Demux/1
  AlphaBetaDot/1 -> Demux2/1
  AngularRates/1 -> Demux3/1
  Demux/3 -> Terminator/1
  Demux/4 -> Terminator1/1
  Demux2/2 -> Terminator2/1
  Demux3/1 -> Terminator3/1
  Demux3/3 -> Terminator4/1
  Sum1/1 -> Cm/1
  Demux1/2 -> Terminator6/1
  2/1 -> Cm*c/(2V)/3
  Wing chord/1 -> Cm*c/(2V)/2
  Sum2/1 -> Cm*c/(2V)/1
  Cmq/1(Coeff) -> Sum2/2
